simulink model "ieee80211n"  (Simulink 6.0)
settings: Solver=VariableStepDiscrete  StartTime=0.0  StopTime=inf  RelTol=1e-3
PreLoadFcn:
  | load IEEE80211n_init;
values from neighbouring files (symbols this model uses):
  params =     [IEEE80211n_init.mat]    (also in IEEE80211n_settings.m = p)
undefined symbols (not defined in the file or in its folder): magnitude
libraries: commblkintrlv2 x196, dspsigops x143, simulink x136, commdigbbndam2 x98, dspmtrx3 x96, dspsigattribs x69, dspstat3 x38, commutil2 x32, commsequence2 x26, commcnvcod2 x10, dspindex x9, dspmlti3 x8
(part 1 of 12)
CloseFcn:
  | IEEE80211n_open_graphics('IEEE80211n/MATLAB graphics', 1)
settings Model: Creator=Martin Clark  LastModifiedBy=Thomas
settings DataIOCC: SaveOutput=off  SaveTime=off  SignalLoggingName=sigsOut
settings OptimizationCC: InlineInvariantSignals=off
settings DebuggingCC: SolverPrmCheckMsg=none
settings HardwareCC: TargetUnknown=on
settings GRTTargetCC: ModelReferenceCompliant=off  MatFileLogging=off

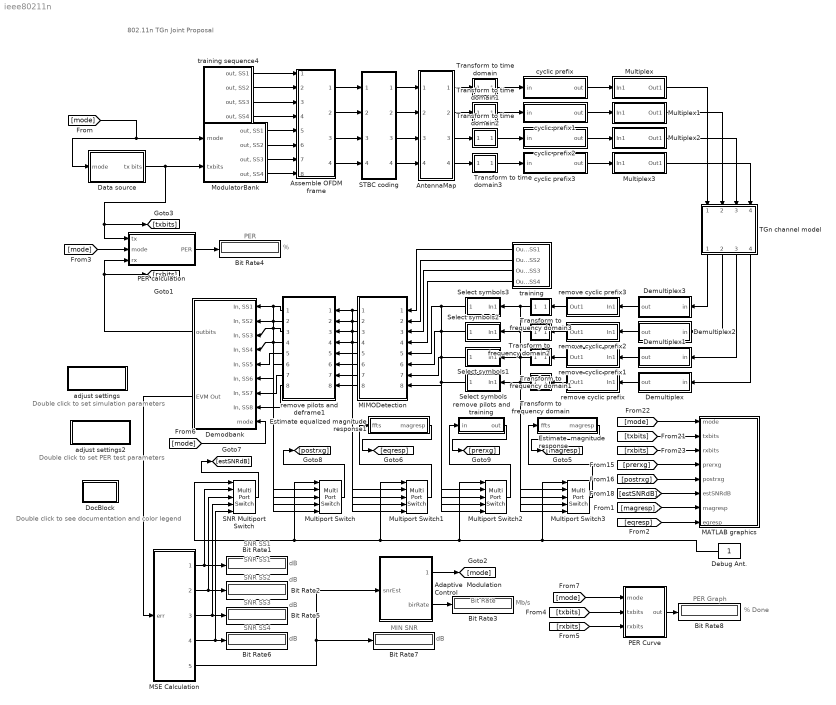
== system ieee80211n ==
  note: 802.11n TGn Joint Proposal
  note: %
  note: SNR SS1
  note: dB
  note: PER
  note: Double click to see
      |  documentation
      | and color legend
  note: Double click to set
      |  simulation parameters
  note: SNR SS2
  note: dB
  note: SNR SS3
  note: dB
  note: SNR SS4
  note: dB
  note: Mb/s
  note: Bit Rate
  note: MIN SNR
  note: dB
  note: SNR SS1
  note: % Done
  note: PER Graph
  note: Double click to set
      |  PER test parameters
  Adaptive  Modulation  Control : Subsystem  mask{thres=[3.5 6.5 9.5 13 17 18.5 20], hyst=2, bitRates=params.NSS * params.bitsPerSymbol * 13}
      mask prompts: thres "Low-SNR thresholds (dB):"; hyst "Hysteresis factor (dB):"; bitRates "Bit rates (Mb/s):"
      mask init:
      | snrUp = [thres inf] + hyst;
      | snrDown = [-inf thres] - hyst;
      mask Display: disp('Adaptive\nModulation\nControl')
  AntennaMap : Subsystem
      mask Display: disp('Antenna\nMap')
  Assemble OFDM frame : Subsystem
      mask Display: disp('Assemble\nOFDM\nFrames')
  Bit Rate{1..8} (8 alike) : Display
  Data source : Subsystem
      mask Display: disp('Variable-Rate\nData source')
  Debug Ant. : Constant  Orientation=left
  Demodbank : Subsystem  Orientation=left
      mask Type: IEEE 802.11n demodulator-decoder bank.
      mask Display: disp('Demodulator\nBank')
  Demultiplex : Subsystem  Orientation=left
      mask Display: disp('Demultiplex\nOFDM Frames')
  Demultiplex1 : Subsystem  Orientation=left
      mask Display: disp('Demultiplex\nOFDM Frames')
  Demultiplex2 : Subsystem  Orientation=left
      mask Display: disp('Demultiplex\nOFDM Frames')
  Demultiplex3 : Subsystem  Orientation=left
      mask Display: disp('Demultiplex\nOFDM Frames')
  DocBlock : Subsystem  mask(DocBlock){ECoderFlag=, DocumentType=Text}
      mask prompts: ECoderFlag "E Coder Flag"; DocumentType "Document Type"
      mask help: Use this block to save long descriptive text with the model. Double-clicking the block will open an editor.
      settings: CopyFcn=docblock('breaklink',gcb);  DeleteFcn=docblock('close_document',gcb);  PreSaveFcn=docblock('save_document',gcb);  OpenFcn=docblock('edit_document',gcb);
      mask StyleString: edit,popup(Text|RTF|HTML)
      mask Display:
      | plot([.8 0 0 1 1 .8 .8 1],[1 1 0 0 .8 1 .8 .8]);
      | text(.5,.5,'DOC','horizontalalignment','center');
  Estimate  magnitude response : Subsystem
      mask Display: disp('Power Spectrum')
  Estimate equalized magnitude response1 : Subsystem
      mask Display: disp('Power Spectrum')
  MATLAB graphics : Subsystem  mask(User-defined graphics.){graphicsName=IEEE80211n_graphics, portNames={'mode', 'txbits', 'rxbits', 'avSNRdB', 'prerxg', 'postrxg', 'estSNRdB', 'magresp', 'eqresp'}, convertMode=structure, extraParams=params}
      mask prompts: graphicsName "Graphics filename (without .fig or .m extension):"; portNames "Port names (cell array):"; convertMode "Data conversion mode:"; extraParams "Additional parameters:"
      mask init:
      | % derive input_names
      | bl = length(gcb);
      | long_names = find_system(gcb,...
      |     'lookundermasks','All',...
      |     'searchdepth', 1,...
      |     'BlockType','Inport');
      | lln = length(long_names);
      | input_names = cell(1, lln);
      | for i=1:lln
      | 	input_names{i}=long_names{i}(bl+2 : end);
      | end
      | 
      | if strcmp(get_param(gcb, 'LinkStatus'), 'resolved')
      | 	set_param(gcb, 'LinkStatus', 'inactive');
      | end
      settings: OpenFcn=IEEE80211n_open_graphics(gcb, 0);
      mask StyleString: edit,edit,popup(cell array|structure),edit
      mask Display: disp('Signal\nVisualization\n\nDouble click to\nopen/close')
  MIMODetection : Subsystem  Orientation=left
      mask Display: disp('MIMO\nDetection')
  MSE Calculation : Subsystem
      mask Display: disp('SNR\nEstimation')
  ModulatorBank : Subsystem
      mask Type: IEEE 802.11n modulator banks for all spatial streams.
      mask Display: disp('Modulator\nBank')
  Multiplex : Subsystem
      mask Display: disp('Multiplex\nOFDM Frames')
  Multiplex1 : Subsystem
      mask Display: disp('Multiplex\nOFDM Frames')
  Multiplex2 : Subsystem
      mask Display: disp('Multiplex\nOFDM Frames')
  Multiplex3 : Subsystem
      mask Display: disp('Multiplex\nOFDM Frames')
  Multiport Switch{,1..3} (4 alike) : MultiPortSwitch  SaturateOnIntegerOverflow=on
  PER Curve : Subsystem
      mask Display: disp('Draw PER\nCurve')
  PER calculation : Subsystem
      mask Display: disp('Packet Error Rate\nCalculation')
  SNR Multiport Switch : MultiPortSwitch  SaturateOnIntegerOverflow=on
  STBC coding : Subsystem
      mask Display: disp('STBC\n+\nCSD1')
  Select symbols : Subsystem  Orientation=left
      mask Display: disp('Remove\nZeros')
  Select symbols1 : Subsystem  Orientation=left
      mask Display: disp('Remove\nZeros')
  Select symbols2 : Subsystem  Orientation=left
      mask Display: disp('Remove\nZeros')
  Select symbols3 : Subsystem  Orientation=left
      mask Display: disp('Remove\nZeros')
  TGn channel model : Subsystem  Orientation=down
      mask Type: Multipath channel model parameters.
      mask Display: disp('TGn Channel\nModel')
  Transform to frequency domain : Subsystem  Orientation=left
      mask Display: disp('FFT')
  Transform to frequency domain1 : Subsystem  Orientation=left
      mask Display: disp('FFT')
  Transform to frequency domain2 : Subsystem  Orientation=left
      mask Display: disp('FFT')
  Transform to frequency domain3 : Subsystem  Orientation=left
      mask Display: disp('FFT')
  Transform to time domain : Subsystem
      mask Display: disp('IFFT')
  Transform to time domain1 : Subsystem
      mask Display: disp('IFFT')
  Transform to time domain2 : Subsystem
      mask Display: disp('IFFT')
  Transform to time domain3 : Subsystem
      mask Display: disp('IFFT')
  adjust settings : Subsystem  Priority=1  mask(IEEE 802.11n model - Settings.){NTX=2, NRX=2, MCS=15, STBC=0, SSpreading=0, Beamform=0, PayloadSize=1000}
      mask prompts: NTX "Number of TX Antennas"; NRX "Number of RX Antennas"; MCS "Modulation/Coding Scheme (MCS)"; STBC "Space-Time Block Coding"; SSpreading "Spatial Spreading"; Beamform "Beamforming"; PayloadSize "Data Payload Size (Bytes)"
      mask help: Parameter settings for IEEE 802.11n model.
      mask init:
      | params = IEEE80211n_settings(...
      | 	NTX, ...
      | 	NRX, ...
      | 	MCS, ...
      | 	SSpreading, ...
      | 	Beamform, ...
      | 	STBC, ...
      |     PayloadSize);
      | 
      | assignin('base', 'params', params);
      mask Help: Parameter settings for IEEE 802.11n model.
      mask Display: disp('Simulation\nSettings')
  adjust settings2 : Subsystem  Priority=1  mask(IEEE 802.11n model - PER Test Settings.){numPkts=1*442, PER_snr=42:-3:18 %[46.2 34.0 26.2 15.7 9.5 5.2]}
      mask prompts: numPkts "Number of Packets / SNR Value"; PER_snr "Vector of SNR Values"
      mask help: PER Test settings for IEEE 802.11n model.
      mask init:
      | per_init(...
      | 	numPkts, ...
      |     PER_snr);
      mask Help: PER Test settings for IEEE 802.11n model.
      mask Display: disp('PER Test\nSettings')
  cyclic prefix : Subsystem
      mask Display: disp('Add CSD2,\nCyclic Prefix')
  cyclic prefix1 : Subsystem
      mask Display: disp('Add CSD2,\nCyclic Prefix')
  cyclic prefix2 : Subsystem
      mask Display: disp('Add CSD2,\nCyclic Prefix')
  cyclic prefix3 : Subsystem
      mask Display: disp('Add CSD2,\nCyclic Prefix')
  remove cyclic prefix : Subsystem  Orientation=left
      mask Display: disp('Remove Cyclic\nPrefix')
  remove cyclic prefix1 : Subsystem  Orientation=left
      mask Display: disp('Remove Cyclic\nPrefix')
  remove cyclic prefix2 : Subsystem  Orientation=left
      mask Display: disp('Remove Cyclic\nPrefix')
  remove cyclic prefix3 : Subsystem  Orientation=left
      mask Display: disp('Remove Cyclic\nPrefix')
  remove pilots and deframe1 : Subsystem  Orientation=left
      mask Display: disp('Disassemble\nOFDM Frames')
  remove pilots and training : Subsystem
      mask Display: disp('Constellation')
  training : Subsystem  Orientation=left
      mask Display: disp('Training')
  training sequence4 : Subsystem
      mask Display: disp('Legacy / HT\nPreamble')
  wires:
  cyclic prefix/1(out) -> Multiplex/1(In1)
  [mode] -> Demodbank/9(mode)
  Demodbank/2(EVM Out) -> MSE Calculation/1(err)
  Data source/1(tx bits) -> PER calculation/1(tx), [txbits], ModulatorBank/2(txbits)
  PER calculation/1(PER) -> Bit Rate4/1
  Transform to time domain/1(out) -> cyclic prefix/1(in)
  Estimate  magnitude response/1(magresp) -> [magresp]
  Estimate equalized magnitude response1/1(magresp) -> [eqresp]
  remove cyclic prefix/1(Out1) -> Transform to frequency domain/1(in)
  MIMODetection/4("out, SS4") -> Multiport Switch1/5, remove pilots and deframe1/4("in, SS4")
  remove pilots and deframe1/4("out, SS4") -> Demodbank/4("In, SS4"), Multiport Switch/5
  Transform to frequency domain/1(out) -> Multiport Switch3/5, Select symbols/1(In1)
  Demultiplex/1(out) -> remove cyclic prefix/1(In1)
  [mode] -> Data source/1(mode), ModulatorBank/1(mode)
  remove pilots and training/1(out) -> [prerxg]
  MSE Calculation/1(estSNR_ss1) -> Bit Rate1/1, SNR Multiport Switch/2
  [mode] -> MATLAB graphics/1(mode)
  [txbits] -> MATLAB graphics/2(txbits)
  [rxbits] -> MATLAB graphics/3(rxbits)
  [prerxg] -> MATLAB graphics/4(prerxg)
  [postrxg] -> MATLAB graphics/5(postrxg)
  [estSNRdB] -> MATLAB graphics/6(estSNRdB)
  [magresp] -> MATLAB graphics/7(magresp)
  [eqresp] -> MATLAB graphics/8(eqresp)
  [mode] -> PER calculation/2(mode)
  training sequence4/1("out, SS1") -> Assemble OFDM frame/1("preamble, SS1")
  ModulatorBank/1("out, SS1") -> Assemble OFDM frame/5("data, SS1")
  training sequence4/2("out, SS2") -> Assemble OFDM frame/2("preamble, SS2")
  training sequence4/3("out, SS3") -> Assemble OFDM frame/3("preamble, SS3")
  training sequence4/4("out, SS4") -> Assemble OFDM frame/4("preamble, SS4")
  ModulatorBank/2("out, SS2") -> Assemble OFDM frame/6("data, SS2")
  ModulatorBank/3("out, SS3") -> Assemble OFDM frame/7("data, SS3")
  ModulatorBank/4("out, SS4") -> Assemble OFDM frame/8("data, SS4")
  Assemble OFDM frame/1("out, SS1") -> STBC coding/1("in, SS1")
  Assemble OFDM frame/2("out, SS2") -> STBC coding/2("in, SS2")
  Assemble OFDM frame/3("out, SS3") -> STBC coding/3("in, SS3")
  Assemble OFDM frame/4("out, SS4") -> STBC coding/4("in, SS4")
  cyclic prefix1/1(out) -> Multiplex1/1(In1)
  Transform to time domain1/1(out) -> cyclic prefix1/1(in)
  cyclic prefix2/1(out) -> Multiplex2/1(In1)
  Transform to time domain2/1(out) -> cyclic prefix2/1(in)
  cyclic prefix3/1(out) -> Multiplex3/1(In1)
  Transform to time domain3/1(out) -> cyclic prefix3/1(in)
  Select symbols/1(Out1) -> Multiport Switch2/5, MIMODetection/8(rxsig4)
  remove cyclic prefix1/1(Out1) -> Transform to frequency domain1/1(in)
  MIMODetection/3("out, SS3") -> remove pilots and deframe1/3("in, SS3"), Multiport Switch1/4
  Transform to frequency domain1/1(out) -> Select symbols1/1(In1), Multiport Switch3/4
  Demultiplex1/1(out) -> remove cyclic prefix1/1(In1)
  remove cyclic prefix2/1(Out1) -> Transform to frequency domain2/1(in)
  MIMODetection/2("out, SS2") -> remove pilots and deframe1/2("in, SS2"), Multiport Switch1/3
  Transform to frequency domain2/1(out) -> Select symbols2/1(In1), Multiport Switch3/3
  Demultiplex2/1(out) -> remove cyclic prefix2/1(In1)
  Select symbols2/1(Out1) -> Multiport Switch2/3, MIMODetection/6(rxsig1)
  remove cyclic prefix3/1(Out1) -> Transform to frequency domain3/1(in)
  MIMODetection/1("out, SS1") -> remove pilots and deframe1/1("in, SS1"), Multiport Switch1/2
  Transform to frequency domain3/1(out) -> Select symbols3/1(In1), Multiport Switch3/2
  Demultiplex3/1(out) -> remove cyclic prefix3/1(In1)
  Select symbols3/1(Out1) -> Multiport Switch2/2, MIMODetection/5(rxsig2)
  remove pilots and deframe1/3("out, SS3") -> Demodbank/3("In, SS3"), Multiport Switch/4
  remove pilots and deframe1/2("out, SS2") -> Demodbank/2("In, SS2"), Multiport Switch/3
  remove pilots and deframe1/1("out, SS1") -> Demodbank/1("In, SS1"), Multiport Switch/2
  TGn channel model/4(Out SS4) -> Demultiplex/1(in)
  TGn channel model/3(Out SS3) -> Demultiplex1/1(in)
  TGn channel model/2(Out SS2) -> Demultiplex2/1(in)
  TGn channel model/1(Out SS1) -> Demultiplex3/1(in)
  Multiplex/1(Out1) -> TGn channel model/1(In SS1)
  Multiplex1/1(Out1) -> TGn channel model/2(In SS2)
  Multiplex2/1(Out1) -> TGn channel model/3(In SS3)
  Multiplex3/1(Out1) -> TGn channel model/4(In SS4)
  AntennaMap/1("out, SS1") -> Transform to time domain/1(in)
  AntennaMap/2("out, SS2") -> Transform to time domain1/1(in)
  AntennaMap/3("out, SS3") -> Transform to time domain2/1(in)
  AntennaMap/4("out, SS4") -> Transform to time domain3/1(in)
  Debug Ant./1 -> Multiport Switch1/1, Multiport Switch2/1, Multiport Switch/1, SNR Multiport Switch/1, Multiport Switch3/1
  Multiport Switch/1 -> [postrxg]
  Multiport Switch1/1 -> Estimate equalized magnitude response1/1(ffts)
  Multiport Switch2/1 -> remove pilots and training/1(in)
  Select symbols1/1(Out1) -> Multiport Switch2/4, MIMODetection/7(rxsig3)
  Multiport Switch3/1 -> Estimate  magnitude response/1(ffts)
  training/1("Out, SS1") -> MIMODetection/1(trainsig1)
  training/2("Out, SS2") -> MIMODetection/2(trainsig2)
  training/3("Out, SS3") -> MIMODetection/3(trainsig3)
  training/4("Out, SS4") -> MIMODetection/4(trainsig4)
  Demodbank/1(outbits) -> PER calculation/3(rx), [rxbits]
  MSE Calculation/2(estSNR_ss2) -> Bit Rate2/1, SNR Multiport Switch/3
  MSE Calculation/3(estSNR_ss3) -> Bit Rate5/1, SNR Multiport Switch/4
  MSE Calculation/4(estSNR_ss4) -> Bit Rate6/1, SNR Multiport Switch/5
  Adaptive  Modulation  Control/2(birRate) -> Bit Rate3/1
  MSE Calculation/5(minSNR) -> Adaptive  Modulation  Control/1(snrEst), Bit Rate7/1
  Adaptive  Modulation  Control/1(modIdx) -> [mode]
  SNR Multiport Switch/1 -> [estSNRdB]
  PER Curve/1(out) -> Bit Rate8/1
  [txbits] -> PER Curve/2(txbits)
  [rxbits] -> PER Curve/3(rxbits)
  [mode] -> PER Curve/1(mode)
  STBC coding/1("out, SS1") -> AntennaMap/1("in, SS1")
  STBC coding/2("out, SS2") -> AntennaMap/2("in, SS2")
  STBC coding/3("out, SS3") -> AntennaMap/3("in, SS3")
  STBC coding/4("out, SS4") -> AntennaMap/4("in, SS4")
  MIMODetection/5("mscale, SS5") -> remove pilots and deframe1/5("mscale in, SS1")
  MIMODetection/6("mscale, SS6") -> remove pilots and deframe1/6("mscale in, SS2")
  MIMODetection/7("mscale, SS7") -> remove pilots and deframe1/7("mscale in, SS3")
  MIMODetection/8("mscale, SS8") -> remove pilots and deframe1/8("mscale in, SS4")
  remove pilots and deframe1/5("mscale out, SS1") -> Demodbank/5("In, SS5")
  remove pilots and deframe1/6("mscale out, SS2") -> Demodbank/6("In, SS6")
  remove pilots and deframe1/7("mscale out, SS3") -> Demodbank/7("In, SS7")
  remove pilots and deframe1/8("mscale out, SS4") -> Demodbank/8("In, SS8")

== system ieee80211n/Adaptive  Modulation  Control ==
  note: inc modIdx by 1
  note: dec modIdx by 1
  note: Bit Rate (Forced)
  note: Bit Rate (Adaptive)
  note: Note: Adaptive rate
      | selection is currently
      | not used
  snrEst : Inport  Port=1  LatchInput=off
  Add1 : Sum  Inputs=+-+  OutDataTypeMode=double  OutScaling=2^-10
  Bit Rate (Adaptive) : IEEE80211a_lib/Select value  vector=bitRates
  Bit Rate (Forced) : IEEE80211a_lib/Select value  vector=bitRates
  Bit Rate1 : Display
  Bit Rate3 : Display
  Delay : dspsigops/Delay  dly_unit=Samples  delay=1  ic_detail=on  dif_ic_for_ch=off  dif_ic_for_dly=on  ic=8  reset_popup=None
  Force Rate : Constant  Value=params.Rate
  Relational Operator : RelationalOperator  Operator=>
  Relational Operator1 : RelationalOperator  Operator=<=
  SNR down threshold : IEEE80211a_lib/Select value  vector=snrDown
  SNR up threshold : Subsystem  AncestorBlock=IEEE80211a_lib/Select value  mask{vector=snrUp}
      mask help: Using MATLAB-style indexing, output value of selected element of vector.
      mask Display: disp('Select\nValue')
  modIdx : Outport
  birRate : Outport  Port=2
  wires:
  snrEst/1 -> Relational Operator/1, Relational Operator1/1
  Relational Operator/1 -> Add1/1
  Relational Operator1/1 -> Add1/2
  SNR up threshold/1(val) -> Relational Operator/2
  SNR down threshold/1 -> Relational Operator1/2
  Add1/1 -> Delay/1
  Bit Rate (Forced)/1 -> birRate/1, Bit Rate3/1
  Force Rate/1 -> modIdx/1, Bit Rate (Forced)/1
  Delay/1 -> Bit Rate (Adaptive)/1, Add1/3, SNR down threshold/1, SNR up threshold/1(idx)
  Bit Rate (Adaptive)/1 -> Bit Rate1/1

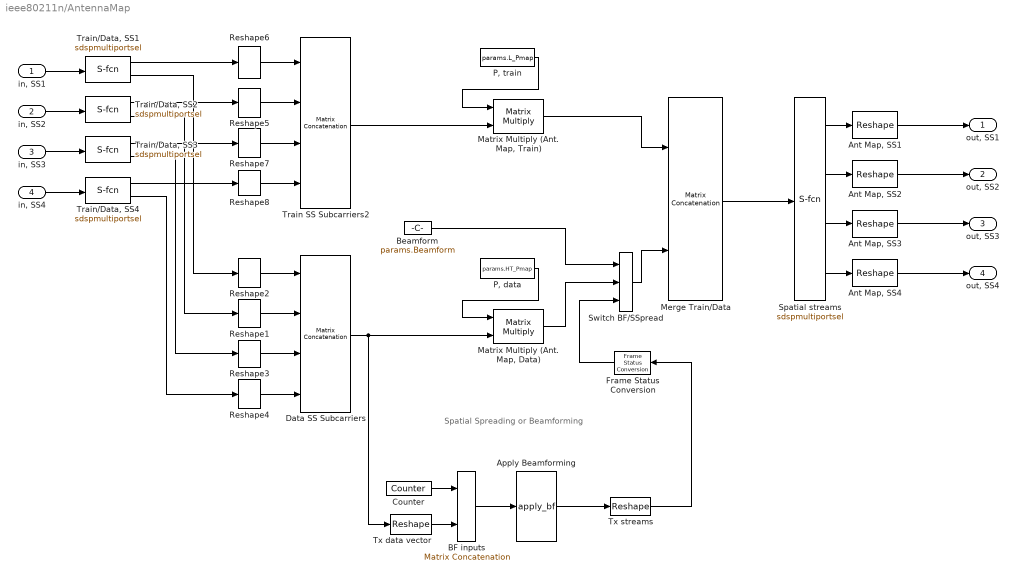
== system ieee80211n/AntennaMap ==
  note: Spatial Spreading
      |
      | or
      |
      | Beamforming
  "in, SS1" : Inport  Port=1  LatchInput=off
  "in, SS2" : Inport  Port=2  LatchInput=off
  "in, SS3" : Inport  Port=3  LatchInput=off
  "in, SS4" : Inport  Port=4  LatchInput=off
  Ant Map, SS{1..4} (4 alike) : simulink/Math Operations/Reshape  OutputDimensionality=Customize  OutputDimensions="[(params.NST+1)  params.OFDMTotSymPerFrame]"
  Apply Beamforming : MATLABFcn  MATLABFcn=apply_bf  OutputDimensions=[4*(params.NST+1)*(params.OFDM_HTSTF_SymPerFrame+params.OFDM_HTLTF_SymPerFrame+params.OFDMSymPerFrame) 1]  Output1D=off
  BF inputs : simulink/Math Operations/Matrix Concatenation  numInports=2  catMethod=Vertical
  Beamform : Constant  Value=params.Beamform
  Counter : dspswit3/Counter  Direction=Up  CountEvent=Free running  CounterSize=32 bits  MaxCount=255  InitialCount=0  Output=Count  HitValue=32  ResetInput=off  SamplesPerFrame=1  Ts=params.minBitPeriod*(params.NSS*params.maxBitsPerBlock)  CntDtype=double  HitDtype=Logical
  Data SS Subcarriers : simulink/Math Operations/Matrix Concatenation  numInports=4  catMethod=Vertical
  Frame Status Conversion : dspsigattribs/Frame Status Conversion  Orientation=left  growRefPort=off  outframe=Sample-based
  "Matrix Multiply (Ant. Map, Data)" : Product  Multiplication=Matrix(*)
  "Matrix Multiply (Ant. Map, Train)" : Product  Multiplication=Matrix(*)
  Merge Train/Data : simulink/Math Operations/Matrix Concatenation  numInports=2  catMethod=Horizontal
  "P, data" : Constant  Value=params.HT_Pmap
  "P, train" : Constant  Value=params.L_Pmap
  Reshape{1..8} (8 alike) : simulink/Math Operations/Reshape  OutputDimensionality=Row vector  OutputDimensions=1600
  Spatial streams : S-Function  AncestorBlock=dspindex/Multiport Selector  FunctionName=sdspmultiportsel  Parameters=rowsOrCols, numOutports, flatIdxVect, flatLenVect, idxErrMode  mask(Multiport Selector){rowsOrCols=Rows, idxCellArray={1 2 3 4}, idxErrMode=Clip Index}
      mask prompts: rowsOrCols "Select:"; idxCellArray "Indices to output:"; idxErrMode "Invalid index:"
      mask help: Output specified rows or columns to one or more output ports. The number of output ports is determined by the number of index vectors, each specified as a separate vector entry in a cell array. Indices are 1-based and need not be unique.
      mask init:
      | [numOutports, flatLenVect, flatIdxVect] = dspblkmultiportsel(idxCellArray);
      mask Help: web(dspbhelp);
      mask StyleString: popup(Rows|Columns),edit,popup(Clip Index|Clip and Warn|Generate Error)
      mask Display: disp(['Select\n' &1]);
  Switch BF/SSpread : MultiPortSwitch  Inputs=2  zeroidx=on  SaturateOnIntegerOverflow=on
  Train SS Subcarriers2 : simulink/Math Operations/Matrix Concatenation  numInports=4  catMethod=Vertical
  "Train/Data, SS1" : S-Function  AncestorBlock=dspindex/Multiport Selector  FunctionName=sdspmultiportsel  Parameters=rowsOrCols, numOutports, flatIdxVect, flatLenVect, idxErrMode  mask(Multiport Selector){rowsOrCols=Columns, idxCellArray={1:params.OFDM_TotPreamblePerFrame-(params.OFDM_HTSTF_SymPerFrame+params.OFDM_HTLTF_SymPerFrame), params.OFDM_TotPreamblePerFrame-(params.OFDM_HTSTF_SymPerFrame+params.OFDM_HTLTF_SymPerFrame)+1:params.OFDMTotSymPerFrame}, idxErrMode=Clip Index}
      mask prompts: rowsOrCols "Select:"; idxCellArray "Indices to output:"; idxErrMode "Invalid index:"
      mask help: Output specified rows or columns to one or more output ports. The number of output ports is determined by the number of index vectors, each specified as a separate vector entry in a cell array. Indices are 1-based and need not be unique.
      mask init:
      | [numOutports, flatLenVect, flatIdxVect] = dspblkmultiportsel(idxCellArray);
      mask Help: web(dspbhelp);
      mask StyleString: popup(Rows|Columns),edit,popup(Clip Index|Clip and Warn|Generate Error)
      mask Display: disp(['Select\n' &1]);
  "Train/Data, SS2" : S-Function  AncestorBlock=dspindex/Multiport Selector  FunctionName=sdspmultiportsel  Parameters=rowsOrCols, numOutports, flatIdxVect, flatLenVect, idxErrMode  mask(Multiport Selector){rowsOrCols=Columns, idxCellArray={1:params.OFDM_TotPreamblePerFrame-(params.OFDM_HTSTF_SymPerFrame+params.OFDM_HTLTF_SymPerFrame), params.OFDM_TotPreamblePerFrame-(params.OFDM_HTSTF_SymPerFrame+params.OFDM_HTLTF_SymPerFrame)+1:params.OFDMTotSymPerFrame}, idxErrMode=Clip Index}
      mask prompts: rowsOrCols "Select:"; idxCellArray "Indices to output:"; idxErrMode "Invalid index:"
      mask help: Output specified rows or columns to one or more output ports. The number of output ports is determined by the number of index vectors, each specified as a separate vector entry in a cell array. Indices are 1-based and need not be unique.
      mask init:
      | [numOutports, flatLenVect, flatIdxVect] = dspblkmultiportsel(idxCellArray);
      mask Help: web(dspbhelp);
      mask StyleString: popup(Rows|Columns),edit,popup(Clip Index|Clip and Warn|Generate Error)
      mask Display: disp(['Select\n' &1]);
  "Train/Data, SS3" : S-Function  AncestorBlock=dspindex/Multiport Selector  FunctionName=sdspmultiportsel  Parameters=rowsOrCols, numOutports, flatIdxVect, flatLenVect, idxErrMode  mask(Multiport Selector){rowsOrCols=Columns, idxCellArray={1:params.OFDM_TotPreamblePerFrame-(params.OFDM_HTSTF_SymPerFrame+params.OFDM_HTLTF_SymPerFrame), params.OFDM_TotPreamblePerFrame-(params.OFDM_HTSTF_SymPerFrame+params.OFDM_HTLTF_SymPerFrame)+1:params.OFDMTotSymPerFrame}, idxErrMode=Clip Index}
      mask prompts: rowsOrCols "Select:"; idxCellArray "Indices to output:"; idxErrMode "Invalid index:"
      mask help: Output specified rows or columns to one or more output ports. The number of output ports is determined by the number of index vectors, each specified as a separate vector entry in a cell array. Indices are 1-based and need not be unique.
      mask init:
      | [numOutports, flatLenVect, flatIdxVect] = dspblkmultiportsel(idxCellArray);
      mask Help: web(dspbhelp);
      mask StyleString: popup(Rows|Columns),edit,popup(Clip Index|Clip and Warn|Generate Error)
      mask Display: disp(['Select\n' &1]);
  "Train/Data, SS4" : S-Function  AncestorBlock=dspindex/Multiport Selector  FunctionName=sdspmultiportsel  Parameters=rowsOrCols, numOutports, flatIdxVect, flatLenVect, idxErrMode  mask(Multiport Selector){rowsOrCols=Columns, idxCellArray={1:params.OFDM_TotPreamblePerFrame-(params.OFDM_HTSTF_SymPerFrame+params.OFDM_HTLTF_SymPerFrame), params.OFDM_TotPreamblePerFrame-(params.OFDM_HTSTF_SymPerFrame+params.OFDM_HTLTF_SymPerFrame)+1:params.OFDMTotSymPerFrame}, idxErrMode=Clip Index}
      mask prompts: rowsOrCols "Select:"; idxCellArray "Indices to output:"; idxErrMode "Invalid index:"
      mask help: Output specified rows or columns to one or more output ports. The number of output ports is determined by the number of index vectors, each specified as a separate vector entry in a cell array. Indices are 1-based and need not be unique.
      mask init:
      | [numOutports, flatLenVect, flatIdxVect] = dspblkmultiportsel(idxCellArray);
      mask Help: web(dspbhelp);
      mask StyleString: popup(Rows|Columns),edit,popup(Clip Index|Clip and Warn|Generate Error)
      mask Display: disp(['Select\n' &1]);
  Tx data vector : simulink/Math Operations/Reshape  OutputDimensionality=Customize  OutputDimensions=[4*(params.NST+1)*(params.OFDM_HTSTF_SymPerFrame+params.OFDM_HTLTF_SymPerFrame+params.OFDMSymPerFrame),1]
  Tx streams : simulink/Math Operations/Reshape  OutputDimensionality=Customize  OutputDimensions=[4, (params.NST+1)*(params.OFDM_HTSTF_SymPerFrame+params.OFDM_HTLTF_SymPerFrame+params.OFDMSymPerFrame)]
  "out, SS1" : Outport
  "out, SS2" : Outport  Port=2
  "out, SS3" : Outport  Port=3
  "out, SS4" : Outport  Port=4
  wires:
  "in, SS1"/1 -> "Train/Data, SS1"/1
  "in, SS2"/1 -> "Train/Data, SS2"/1
  "in, SS3"/1 -> "Train/Data, SS3"/1
  "in, SS4"/1 -> "Train/Data, SS4"/1
  Reshape2/1 -> Data SS Subcarriers/1
  Reshape1/1 -> Data SS Subcarriers/2
  Reshape3/1 -> Data SS Subcarriers/3
  Reshape4/1 -> Data SS Subcarriers/4
  Data SS Subcarriers/1 -> "Matrix Multiply (Ant. Map, Data)"/2, Tx data vector/1
  "P, data"/1 -> "Matrix Multiply (Ant. Map, Data)"/1
  "Train/Data, SS4"/2 -> Reshape4/1
  "Train/Data, SS3"/2 -> Reshape3/1
  "Train/Data, SS2"/2 -> Reshape1/1
  "Train/Data, SS1"/2 -> Reshape2/1
  Reshape6/1 -> Train SS Subcarriers2/1
  Reshape5/1 -> Train SS Subcarriers2/2
  Reshape7/1 -> Train SS Subcarriers2/3
  Reshape8/1 -> Train SS Subcarriers2/4
  Train SS Subcarriers2/1 -> "Matrix Multiply (Ant. Map, Train)"/2
  "P, train"/1 -> "Matrix Multiply (Ant. Map, Train)"/1
  "Train/Data, SS1"/1 -> Reshape6/1
  "Train/Data, SS2"/1 -> Reshape5/1
  "Train/Data, SS3"/1 -> Reshape7/1
  "Train/Data, SS4"/1 -> Reshape8/1
  "Matrix Multiply (Ant. Map, Train)"/1 -> Merge Train/Data/1
  "Matrix Multiply (Ant. Map, Data)"/1 -> Switch BF/SSpread/2
  Merge Train/Data/1 -> Spatial streams/1
  "Ant Map, SS1"/1 -> "out, SS1"/1
  "Ant Map, SS2"/1 -> "out, SS2"/1
  "Ant Map, SS3"/1 -> "out, SS3"/1
  "Ant Map, SS4"/1 -> "out, SS4"/1
  Spatial streams/1 -> "Ant Map, SS1"/1
  Spatial streams/2 -> "Ant Map, SS2"/1
  Spatial streams/3 -> "Ant Map, SS3"/1
  Spatial streams/4 -> "Ant Map, SS4"/1
  Apply Beamforming/1 -> Tx streams/1
  Switch BF/SSpread/1 -> Merge Train/Data/2
  Beamform/1 -> Switch BF/SSpread/1
  Tx data vector/1 -> BF inputs/2
  Tx streams/1 -> Frame Status Conversion/1
  Frame Status Conversion/1 -> Switch BF/SSpread/3
  BF inputs/1 -> Apply Beamforming/1
  Counter/1 -> BF inputs/1

== system ieee80211n/Assemble OFDM frame ==
  "preamble, SS1" : Inport  Port=1  LatchInput=off
  "preamble, SS2" : Inport  Port=2  LatchInput=off
  "preamble, SS3" : Inport  Port=3  LatchInput=off
  "preamble, SS4" : Inport  Port=4  LatchInput=off
  "data, SS1" : Inport  Port=5  LatchInput=off
  "data, SS2" : Inport  Port=6  LatchInput=off
  "data, SS3" : Inport  Port=7  LatchInput=off
  "data, SS4" : Inport  Port=8  LatchInput=off
  Prepend training seq{,1..3} (4 alike) : simulink/Math Operations/Matrix Concatenation  numInports=2  catMethod=Horizontal
  "out, SS1" : Outport
  "out, SS2" : Outport  Port=2
  "out, SS3" : Outport  Port=3
  "out, SS4" : Outport  Port=4
  wires:
  "preamble, SS1"/1 -> Prepend training seq/1
  Prepend training seq/1 -> "out, SS1"/1
  "preamble, SS2"/1 -> Prepend training seq1/1
  Prepend training seq1/1 -> "out, SS2"/1
  "preamble, SS3"/1 -> Prepend training seq2/1
  Prepend training seq2/1 -> "out, SS3"/1
  "preamble, SS4"/1 -> Prepend training seq3/1
  Prepend training seq3/1 -> "out, SS4"/1
  "data, SS1"/1 -> Prepend training seq/2
  "data, SS2"/1 -> Prepend training seq1/2
  "data, SS3"/1 -> Prepend training seq2/2
  "data, SS4"/1 -> Prepend training seq3/2

== system ieee80211n/Data source ==
  mode : Inport  Port=1  LatchInput=off
  Binary source : Subsystem  TreatAsAtomicUnit=on  mask{sample_time=params.minBitPeriod, samp_per_frame=params.nSource}
      mask prompts: sample_time "Sample time:"; samp_per_frame "Samples per frame:"
      mask help: Enabled binary data source
  Buffer : dspbuff3/Buffer  N=params.NSS*params.maxBitsPerBlock  V=0  ic=0
  Source enable : Subsystem
  tx bits : Outport
  wires:
  Binary source/1(data out) -> Buffer/1
  Buffer/1 -> tx bits/1
  mode/1 -> Source enable/1(mode)
  Source enable/1(enable) -> Binary source/Enable

== system ieee80211n/Demodbank ==
  "In, SS1" : Inport  Orientation=left  Port=1  LatchInput=off
  "In, SS2" : Inport  Orientation=left  Port=2  LatchInput=off
  "In, SS3" : Inport  Orientation=left  Port=3  LatchInput=off
  "In, SS4" : Inport  Orientation=left  Port=4  LatchInput=off
  "In, SS5" : Inport  Orientation=left  Port=5  LatchInput=off
  "In, SS6" : Inport  Orientation=left  Port=6  LatchInput=off
  "In, SS7" : Inport  Orientation=left  Port=7  LatchInput=off
  "In, SS8" : Inport  Orientation=left  Port=8  LatchInput=off
  mode : Inport  Orientation=left  Port=9  LatchInput=off
  DecodeBankViterbi : Subsystem  Orientation=left  mask(IEEE 802.11a demodulator-decoder bank.){nSymbolsPerFrame=params.NSS*params.numTxSymbols, vtbd_set=params.vtbd_set}
      mask prompts: nSymbolsPerFrame "Number of symbols per frame:"; vtbd_set "vtbd set"
      mask init:
      | numModulators = 8;
      | modulation = {'BPSK' 'QPSK' 'QPSK' '16-QAM' '16-QAM' '64-QAM' '64-QAM' '64-QAM'};
      | code = {'1/2' '1/2' '3/4' '1/2' '3/4' '2/3' '3/4' '5/6'};
      | 
      | % modulation-specific
      | TS1 = 'poly2trellis(7, [171 133])';
      | TS2 = 'poly2trellis(7, [133 171])';
      | trellisStructure = {TS1 TS1 TS1 TS1 TS1 TS2 TS2 TS2};
      | 
      | % code-specific
      | PV = {'[1]', '[1 1 1 0].''', '[1 1 1 0 0 1].''', '[1]', '[1 1 1 0 0 1 1 0 0 1].'''};
      | punctureVector = {PV{1} PV{1} PV{3} PV{1} PV{3} PV{2} PV{3} PV{5}};
      | 
      | for n = 1:numModulators
      |     blk = [gcb '/Demodulator ' num2str(n)];
      |     set_param(blk, 'numSymbols', num2str(nSymbolsPerFrame));
      |     set_param(blk, 'modulation', modulation{n});
      |     set_param(blk, 'code', code{n});
      |     set_param(blk, 'trellisStructure', trellisStructure{n});
      |     set_param(blk, 'punctureVector', punctureVector{n});
      | end
      mask Display: disp('Decode Bank\n(Viterbi)')
  Demod_ss1 : Subsystem  Orientation=left  mask(IEEE 802.11a demodulator-decoder bank.){nSymbolsPerFrame=params.numTxSymbols, vtbd_set=params.vtbd_set}
      mask prompts: nSymbolsPerFrame "Number of symbols per frame:"; vtbd_set "vtbd set"
      mask init: same as ieee80211n/Demodbank/DecodeBankViterbi
      mask Display: disp('Demodulator\nBank\nSS1')
  Demod_ss2 : Subsystem  Orientation=left  mask(IEEE 802.11a demodulator-decoder bank.){nSymbolsPerFrame=params.numTxSymbols, vtbd_set=params.vtbd_set}
      mask prompts: nSymbolsPerFrame "Number of symbols per frame:"; vtbd_set "vtbd set"
      mask init:
      | numModulators = 8;
      | modulation = {'BPSK' 'QPSK' 'QPSK' '16-QAM' '16-QAM' '64-QAM' '64-QAM' '64-QAM'};
      | code = {'1/2' '1/2' '3/4' '1/2' '3/4' '2/3' '3/4' '5/6'};
      | 
      | % modulation-specific
      | TS1 = 'poly2trellis(7, [171 133])';
      | TS2 = 'poly2trellis(7, [133 171])';
      | trellisStructure = {TS1 TS1 TS1 TS1 TS1 TS2 TS2 TS2};
      | 
      | % code-specific
      | PV = {'[1]', '[1 1 1 0].''', '[1 1 1 0 0 1].''', '[1]', '[1 1 1 0 0 1 1 0 0 1].'''};
      | punctureVector = {PV{1} PV{1} PV{3} PV{1} PV{3} PV{2} PV{3} PV{5}};
      | 
      | for n = 1:numModulators
      |     blk = [gcb '/Demodulator ' num2str(n)];
      |     set_param(blk, 'numSymbols', num2str(nSymbolsPerFrame));
      |     set_param(blk, 'modulation', modulation{n});
      |     set_param(blk, 'code', code{n});
      |     set_param(blk, 'trellisStructure', trellisStructure{n});
      |     set_param(blk, 'punctureVector', punctureVector{n});
      | end
      mask Display: disp('Demodulator\nBank\nSS2')
  Demod_ss3 : Subsystem  Orientation=left  mask(IEEE 802.11a demodulator-decoder bank.){nSymbolsPerFrame=params.numTxSymbols, vtbd_set=params.vtbd_set}
      mask prompts: nSymbolsPerFrame "Number of symbols per frame:"; vtbd_set "vtbd set"
      mask init: same as ieee80211n/Demodbank/Demod_ss2
      mask Display: disp('Demodulator\nBank\nSS3')
  Demod_ss4 : Subsystem  Orientation=left  mask(IEEE 802.11a demodulator-decoder bank.){nSymbolsPerFrame=params.numTxSymbols, vtbd_set=params.vtbd_set}
      mask prompts: nSymbolsPerFrame "Number of symbols per frame:"; vtbd_set "vtbd set"
      mask init: same as ieee80211n/Demodbank/Demod_ss2
      mask Display: disp('Demodulator\nBank\nSS4')
  EVM streams : simulink/Math Operations/Matrix Concatenation  Orientation=left  numInports=4  catMethod=Horizontal
  Nss : Constant  Orientation=left  Value=params.NSS
  Parsing Input : simulink/Math Operations/Matrix Concatenation  Orientation=left  numInports=11  catMethod=Vertical
  Reverse Spatial Parsing : MATLABFcn  Orientation=left  MATLABFcn=rev_spatial_parse  OutputDimensions=[2*4*params.maxTxBitsPerBlock 1]  Output1D=off
  blksize : Constant  Orientation=left  Value=params.maxTxBitsPerBlock
  outbits : Outport  Orientation=left
  EVM Out : Outport  Orientation=left  Port=2
  wires:
  Demod_ss1/1(rxbits) -> Parsing Input/4
  Demod_ss2/1(rxbits) -> Parsing Input/5
  Demod_ss3/1(rxbits) -> Parsing Input/6
  Demod_ss4/1(rxbits) -> Parsing Input/7
  Demod_ss4/2(EVM) -> EVM streams/4
  "In, SS1"/1 -> Demod_ss1/2(sig)
  "In, SS2"/1 -> Demod_ss2/2(sig)
  "In, SS3"/1 -> Demod_ss3/2(sig)
  "In, SS4"/1 -> Demod_ss4/2(sig)
  mode/1 -> Demod_ss2/1(mode), Demod_ss1/1(mode), Parsing Input/1, Demod_ss3/1(mode), Demod_ss4/1(mode), DecodeBankViterbi/1(mode)
  Demod_ss1/2(EVM) -> EVM streams/1
  Reverse Spatial Parsing/1 -> DecodeBankViterbi/2(sig)
  DecodeBankViterbi/1(rxbits) -> outbits/1
  Nss/1 -> Parsing Input/2
  blksize/1 -> Parsing Input/3
  Parsing Input/1 -> Reverse Spatial Parsing/1
  EVM streams/1 -> EVM Out/1
  Demod_ss2/2(EVM) -> EVM streams/2
  Demod_ss3/2(EVM) -> EVM streams/3
  "In, SS5"/1 -> Demod_ss1/3(mscale)
  "In, SS6"/1 -> Demod_ss2/3(mscale)
  "In, SS7"/1 -> Demod_ss3/3(mscale)
  "In, SS8"/1 -> Demod_ss4/3(mscale)
  Demod_ss1/3(mscale out) -> Parsing Input/8
  Demod_ss2/3(mscale out) -> Parsing Input/9
  Demod_ss3/3(mscale out) -> Parsing Input/10
  Demod_ss4/3(mscale out) -> Parsing Input/11

== system ieee80211n/Demultiplex ==
  in : Inport  Port=1  LatchInput=off
  Demultiplex : simulink/Math Operations/Reshape  OutputDimensionality=Customize  OutputDimensions="[params.NFFT2  params.OFDMTotSymPerFrame]"
  out : Outport
  wires:
  Demultiplex/1 -> out/1
  in/1 -> Demultiplex/1

== system ieee80211n/Demultiplex1 ==
  in : Inport  Port=1  LatchInput=off
  Demultiplex : simulink/Math Operations/Reshape  OutputDimensionality=Customize  OutputDimensions="[params.NFFT2  params.OFDMTotSymPerFrame]"
  out : Outport
  wires:
  Demultiplex/1 -> out/1
  in/1 -> Demultiplex/1

== system ieee80211n/Demultiplex2 ==
  in : Inport  Port=1  LatchInput=off
  Demultiplex : simulink/Math Operations/Reshape  OutputDimensionality=Customize  OutputDimensions="[params.NFFT2  params.OFDMTotSymPerFrame]"
  out : Outport
  wires:
  Demultiplex/1 -> out/1
  in/1 -> Demultiplex/1

== system ieee80211n/Demultiplex3 ==
  in : Inport  Port=1  LatchInput=off
  Demultiplex : simulink/Math Operations/Reshape  OutputDimensionality=Customize  OutputDimensions="[params.NFFT2  params.OFDMTotSymPerFrame]"
  out : Outport
  wires:
  Demultiplex/1 -> out/1
  in/1 -> Demultiplex/1

== system ieee80211n/DocBlock ==
  EmptySubsystem : Subsystem

== system ieee80211n/Estimate  magnitude response ==
  ffts : Inport  Port=1  LatchInput=off
  Math Function : Math  Operator=magnitude^2  SaturateOnIntegerOverflow=on
  Mean : dspstat3/Mean  DialogController=dspDDGCreate  DialogControllerArgs=DataTag1  run=off  reset_popup=None  roundingMode=Floor  overflowMode=off
  Transpose : dspmtrx3/Transpose  Hermitian=off  overflowFlag=on
  Transpose1 : dspmtrx3/Transpose  Hermitian=off  overflowFlag=on
  dB Conversion : dspmathops/dB Conversion  dBtype=dB  intype=Power  R=1  fuzz=on
  magresp : Outport
  wires:
  dB Conversion/1 -> magresp/1
  Transpose1/1 -> dB Conversion/1
  Transpose/1 -> Mean/1
  Mean/1 -> Transpose1/1
  ffts/1 -> Math Function/1
  Math Function/1 -> Transpose/1

== system ieee80211n/Estimate equalized magnitude response1 ==
  ffts : Inport  Port=1  LatchInput=off
  Constant : Constant  Value=NaN
  Math Function : Math  Operator=magnitude^2  SaturateOnIntegerOverflow=on
  Matrix Concatenation : simulink/Math Operations/Matrix Concatenation  numInports=3  catMethod=Vertical
  Mean : dspstat3/Mean  DialogController=dspDDGCreate  DialogControllerArgs=DataTag2  run=off  reset_popup=None  roundingMode=Floor  overflowMode=off
  Transpose : dspmtrx3/Transpose  Hermitian=off  overflowFlag=on
  Transpose1 : dspmtrx3/Transpose  Hermitian=off  overflowFlag=on
  dB Conversion1 : dspmathops/dB Conversion  dBtype=dB  intype=Power  R=1  fuzz=on
  dB Conversion2 : dspmathops/dB Conversion  dBtype=dB  intype=Power  R=1  fuzz=on
  negative frequencies : Selector  Elements=[1:params.NST/2]  InputPortWidth=params.NST
  positive frequencies : Selector  Elements=params.NST/2+1:params.NST  InputPortWidth=params.NST
  magresp : Outport
  wires:
  Constant/1 -> Matrix Concatenation/2
  Matrix Concatenation/1 -> magresp/1
  dB Conversion2/1 -> Matrix Concatenation/3
  positive frequencies/1 -> dB Conversion2/1
  dB Conversion1/1 -> Matrix Concatenation/1
  negative frequencies/1 -> dB Conversion1/1
  Transpose1/1 -> positive frequencies/1, negative frequencies/1
  Transpose/1 -> Mean/1
  Mean/1 -> Transpose1/1
  ffts/1 -> Math Function/1
  Math Function/1 -> Transpose/1

== system ieee80211n/MATLAB graphics ==
  mode : Inport  Port=1  LatchInput=off
  txbits : Inport  Port=2  LatchInput=off
  rxbits : Inport  Port=3  LatchInput=off
  prerxg : Inport  Port=4  LatchInput=off
  postrxg : Inport  Port=5  LatchInput=off
  estSNRdB : Inport  Port=6  LatchInput=off
  magresp : Inport  Port=7  LatchInput=off
  eqresp : Inport  Port=8  LatchInput=off
  Transform data : Subsystem
      mask Display: disp('Transform\nData')
  append1 : Subsystem
      mask Display: disp('Append\nSize')
  append2 : Subsystem
      mask Display: disp('Append\nSize')
  append3 : Subsystem
      mask Display: disp('Append\nSize')
  append5 : Subsystem
      mask Display: disp('Append\nSize')
  append6 : Subsystem
      mask Display: disp('Append\nSize')
  append7 : Subsystem
      mask Display: disp('Append\nSize')
  append8 : Subsystem
      mask Display: disp('Append\nSize')
  append9 : Subsystem
      mask Display: disp('Append\nSize')
  concat : simulink/Math Operations/Matrix Concatenation  numInports=8  catMethod=Vertical
  graphics : S-Function  FunctionName=IEEE80211n_udg  Parameters={input_names, extraParams}
  wires:
  eqresp/1 -> append9/1(in)
  magresp/1 -> append8/1(in)
  estSNRdB/1 -> append7/1(in)
  postrxg/1 -> append6/1(in)
  prerxg/1 -> append5/1(in)
  rxbits/1 -> append3/1(in)
  txbits/1 -> append2/1(in)
  Transform data/1(out) -> graphics/1
  concat/1 -> Transform data/1(in)
  mode/1 -> append1/1(in)
  append1/1(out) -> concat/1
  append2/1(out) -> concat/2
  append3/1(out) -> concat/3
  append9/1(out) -> concat/8
  append8/1(out) -> concat/7
  append7/1(out) -> concat/6
  append6/1(out) -> concat/5
  append5/1(out) -> concat/4
